simulink model "pcss_example_2"  (R2021b)
settings: Solver=ode45  StartTime=0.0  StopTime=3000  FixedStep=0.1  MaxStep=0.1  MinStep=0.001  RelTol=1e-3  EnableMultiTasking=on
libraries: mpclib x1, simulink_need_slupdate x1
settings Model: Creator=t1714  LastModifiedBy=t1714
settings DataIOCC: Decimation=5  MaxDataPoints=100  SaveFormat=StructureWithTime  SignalLoggingSaveFormat=ModelDataLogs  SignalLogging=off  SaveTime=off  ReturnWorkspaceOutputs=off
settings OptimizationCC: InitFltsAndDblsToZero=on  LifeSpan=inf
settings DebuggingCC: SaveWithParameterizedLinksMsg=none  UnderspecifiedInitializationDetection=Classic  MergeDetectMultiDrivingBlocksExec=none  SignalResolutionControl=TryResolveAllWithWarning  MultiTaskDSMMsg=warning  MultiTaskCondExecSysMsg=none  FcnCallInpInsideContextMsg=warning  SFUnexpectedBacktrackingDiag=warning  SFNoUnconditionalDefaultTransitionDiag=warning  SFExecutionAtInitializationDiag=none  SFMachineParentedDataDiag=warning  ArithmeticOperatorsInVariantConditions=warning
settings HardwareCC: ProdBitPerPointer=32  ProdBitPerSizeT=32  ProdBitPerPtrDiffT=32  ProdLargestAtomicFloat=None  ProdIntDivRoundTo=Undefined  ProdEndianess=Unspecified  ProdWordSize=32  ProdHWDeviceType=32-bit Generic
settings ModelReferenceCC: PropagateSignalLabelsOutOfModel=off
settings SFSimCC: SimParseCustomCode=off
settings CodeAppCC: StateflowObjectComments=on
settings GRTTargetCC: TargetFcnLib=ansi_tfl_tmw.mat  TargetLangStandard=C89/C90 (ANSI)  CombineOutputUpdateFcns=off  GRTInterface=on
settings ConfigComp: CovMetricSettings=dw  CovSaveCumulativeToWorkspaceVar=on  CovSaveSingleToWorkspaceVar=on

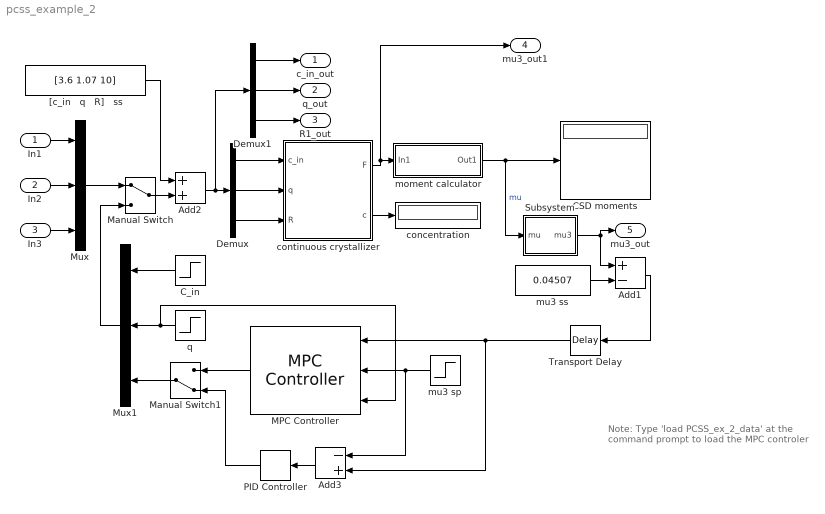
== system pcss_example_2 ==
  note: Note: Type 'load PCSS_ex_2_data' at the
      |   command prompt to load the MPC controler
  In1 : Inport  Interpolate=off
  In2 : Inport  Port=2  Interpolate=off
  In3 : Inport  Port=3  Interpolate=off
  Add1 : Sum  Inputs=+-
  Add2 : Sum
  Add3 : Sum  Inputs=-+
  CSD moments : Display
  C_in : Step  Time=500  After=0  SampleTime=0
  Demux : Demux  Outputs=3
  Demux1 : Demux  Outputs=3
  MPC Controller : mpclib/MPC Controller  mpcobj=PCSS_ex_2_MPC  x0=[]  is_multiple=0  enable_value=0  return_u0=off  updateMPCinCallerWorkspace=on  md_inport=on  mv_inport=off  uref_inport=off  return_cost=off  return_mvseq=off  return_qpstatus=off  return_xseq=off  return_state=off  return_ovseq=off  state_inport=off  umin_inport=off  umax_inport=off  ymin_inport=off  ymax_inport=off  cc_inport=off  ywt_inport=off  uwt_inport=off  duwt_inport=off  rhoeps_inport=off  pm_inport=off  MaximumP=10  HorizonChoice=FixedHorizon  n_ts=50  n_p=10  n_mv=1  n_md=1  n_ud=1  n_mo=1  n_uo=0  BlockDataType=double  SampleTimeInherited=off  switch_inport=off
  Manual Switch : ManualSwitch
  Manual Switch1 : ManualSwitch  CurrentSetting=0
  Mux : Mux  Inputs=3
  Mux1 : Mux  Inputs=3
  PID Controller : simulink_need_slupdate/PID Controller  P=1.4  I=1.2  D=0
  Subsystem : Subsystem
  Transport Delay : TransportDelay  DelayTime=2
  "[c_in   q   R]   ss" : Constant  Value=[3.6 1.07 10]
  concentration : Display
  continuous crystallizer : Subsystem
      mask Display:
      | disp('PCSS')
      | port_label('input',1,'c_in')
      | port_label('input',2,'q')
      | port_label('input',3,'R')
      | port_label('output',1,'F')
      | port_label('output',2,'c')
  moment calculator : Subsystem  mask{dL='pcss_ex_2', mucalc=[0,1,2,3], mu_plot=[0 3], gf=[]}
      mask prompts: dL "What is the value of dL?"; mucalc "Which moments should be calculated and output?"; mu_plot "Which moments should be graphed?"; gf "How often should the graph be updated?"
      mask Display:
      | port_label('input', 1, 'F')
      | port_label('output', 1, 'mu')
  mu3 sp : Step  Time=500  After=0  SampleTime=0
  mu3 ss : Constant  Value=0.04507
  q : Step  Time=500  After=0  SampleTime=0
  c_in_out : Outport
  q_out : Outport  Port=2
  R1_out : Outport  Port=3
  mu3_out1 : Outport  Port=4
  mu3_out : Outport  Port=5
  wires:
  moment calculator/1(Out1) -> CSD moments/1, Subsystem/1(mu)  "mu"
  continuous crystallizer/1(F) -> mu3_out1/1, moment calculator/1(In1)
  continuous crystallizer/2(c) -> concentration/1
  In3/1 -> Mux/3
  In2/1 -> Mux/2
  In1/1 -> Mux/1
  Demux/1 -> continuous crystallizer/1(c_in)
  Demux/2 -> continuous crystallizer/2(q)
  Demux/3 -> continuous crystallizer/3(R)
  Add2/1 -> Demux/1, Demux1/1
  "[c_in   q   R]   ss"/1 -> Add2/1
  Subsystem/1(mu3) -> Add1/1, mu3_out/1
  mu3 ss/1 -> Add1/2
  Manual Switch/1 -> Add2/2
  Mux/1 -> Manual Switch/1
  C_in/1 -> Mux1/1
  Mux1/1 -> Manual Switch/2
  mu3 sp/1 -> Add3/1, MPC Controller/2
  q/1 -> Mux1/2, MPC Controller/3
  Manual Switch1/1 -> Mux1/3
  MPC Controller/1 -> Manual Switch1/1
  PID Controller/1 -> Manual Switch1/2
  Add3/1 -> PID Controller/1
  Add1/1 -> Transport Delay/1
  Demux1/1 -> c_in_out/1
  Demux1/2 -> q_out/1
  Demux1/3 -> R1_out/1
  Transport Delay/1 -> Add3/2, MPC Controller/1

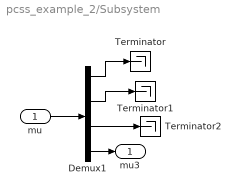
== system pcss_example_2/Subsystem ==
  mu : Inport
  Demux1 : Demux
  Terminator : Terminator
  Terminator1 : Terminator
  Terminator2 : Terminator
  mu3 : Outport
  wires:
  Demux1/1 -> Terminator/1
  Demux1/2 -> Terminator1/1
  Demux1/3 -> Terminator2/1
  mu/1 -> Demux1/1
  Demux1/4 -> mu3/1

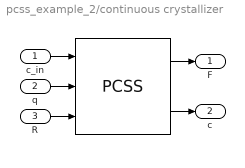
== system pcss_example_2/continuous crystallizer ==
  c_in : Inport
  q : Inport  Port=2
  R : Inport  Port=3
  " " : M-S-Function  FunctionName=PCSS  Parameters='pcss_ex_2'
  F : Outport
  c : Outport  Port=2
  wires:
  c_in/1 -> " "/1
  " "/1 -> F/1
  q/1 -> " "/2
  " "/2 -> c/1
  R/1 -> " "/3

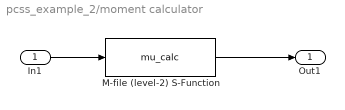
== system pcss_example_2/moment calculator ==
  In1 : Inport
  M-file (level-2) S-Function : M-S-Function  FunctionName=mu_calc  Parameters=dL,mucalc,mu_plot,gf
  Out1 : Outport
  wires:
  M-file (level-2) S-Function/1 -> Out1/1
  In1/1 -> M-file (level-2) S-Function/1
